simulink model "turbocarsim"  (Simulink 5.1)
settings: Solver=ode45  StartTime=0.0  StopTime=20  RelTol=1e-3
libraries: mpt_sim x2
settings Model: LastModifiedBy=michal  BooleanDataType=on

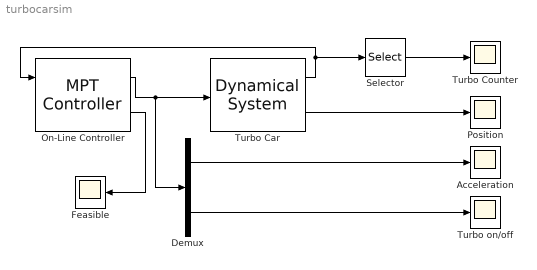
== system turbocarsim ==
  Acceleration : Scope
      settings: TimeRange=20  YMin=-1  YMax=1.5  SaveToWorkspace=off  LimitDataPoints=on  MaxDataPoints=5000
  Demux : Demux  Outputs=2  BusSelectionMode=off
  Feasible : Scope
      settings: TimeRange=20  YMin=0  YMax=1  SaveToWorkspace=off  SaveName=ScopeData4  LimitDataPoints=on  MaxDataPoints=5000
  On-Line Controller : mpt_sim/MPT Controller  ctrl=onlc  Ts=[]  infbreak=on
  Position : Scope
      settings: TimeRange=20  YMin=0  YMax=20  SaveToWorkspace=off  SaveName=ScopeData  LimitDataPoints=on  MaxDataPoints=5000
  Selector : Selector  InputType=Vector  ElementSrc=Internal  Elements=3  RowSrc=Internal  Rows=1  ColumnSrc=Internal  Columns=1  InputPortWidth=3
  Turbo Car : mpt_sim/Dynamical System  sysStruct=sysStruct  x0=[20;0;5]  Ts=[]  constr=on
  Turbo Counter : Scope
      settings: TimeRange=auto  YMin=-5  YMax=5  SaveToWorkspace=off  SaveName=ScopeData3  LimitDataPoints=on  MaxDataPoints=5000
  Turbo on/off : Scope
      settings: TimeRange=20  YMin=0  YMax=1  SaveToWorkspace=off  SaveName=ScopeData2  LimitDataPoints=on  MaxDataPoints=5000
  wires:
  On-Line Controller/1 -> Turbo Car/1, Demux/1
  Turbo Car/1 -> On-Line Controller/1, Selector/1
  Turbo Car/2 -> Position/1
  Demux/1 -> Acceleration/1
  Demux/2 -> Turbo on/off/1
  Selector/1 -> Turbo Counter/1
  On-Line Controller/2 -> Feasible/1
